simulink model "untitled"  (R2017a)
settings: Solver=VariableStepAuto  StartTime=0.0  StopTime=10.0  RelTol=1e-3
settings Model: Creator=frede  LastModifiedBy=frede

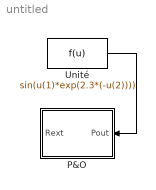
== system untitled ==
  P&O : MATLAB Function  TreatAsAtomicUnit=on
  Unité : Fcn  Expr=sin(u(1)*exp(2.3*(-u(2))))
  wires:
  Unité/1 -> P&O/1(Pout)

== matlab function untitled/P&O ==
  data: Pout input; Rext output
function Rext = fcn(Pout)

Rext = Pout;
